simulink model "dvbs2hdlTransmitterCore"  (R2024b)
settings: Solver=FixedStepDiscrete  StartTime=0.0  StopTime=0  RelTol=1e-3
libraries: hdlsllib x105, simulink x41, dspsigops x7, commseqgen3 x5, whdlutilities x5, commhdlcrc x2, dsphdlfiltering2 x1, whdlmod x1
(part 3 of 5)

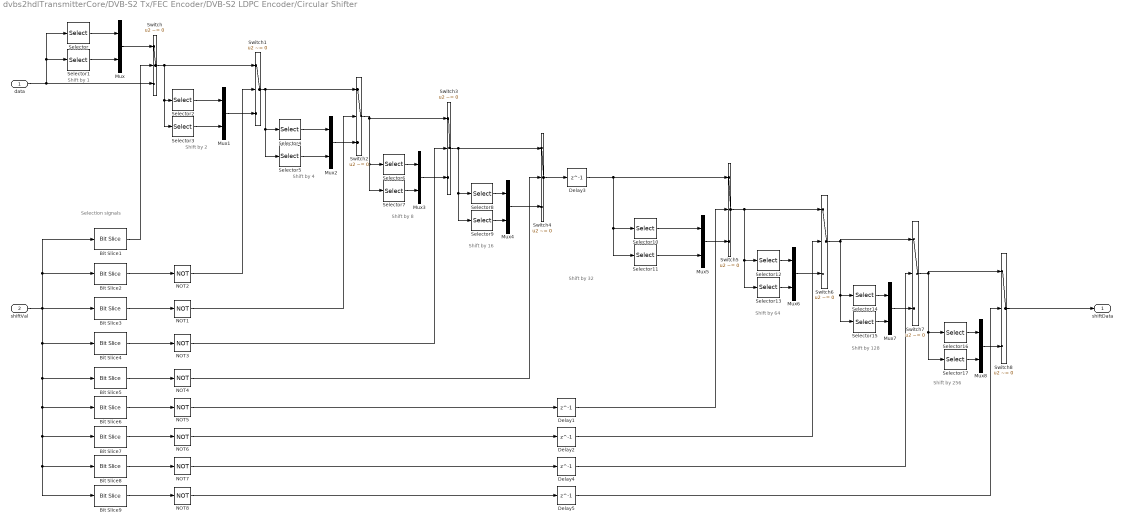
== system dvbs2hdlTransmitterCore/DVB-S2 Tx/FEC Encoder/DVB-S2 LDPC Encoder/Circular Shifter ==
  note: Shift by 256
  note: Shift by 128
  note: Shift by 64
  note: Shift by 32
  note: Shift by 16
  note: Shift by 8
  note: Shift by 4
  note: Shift by 2
  note: Shift by 1
  note: Selection signals
  data : Inport
  shiftVal : Inport  Port=2
  Bit Slice1 : hdlsllib/Logic and Bit Operations/Bit Slice  lidx=0  ridx=0
  Bit Slice2 : hdlsllib/Logic and Bit Operations/Bit Slice  lidx=1  ridx=1
  Bit Slice3 : hdlsllib/Logic and Bit Operations/Bit Slice  lidx=2  ridx=2
  Bit Slice4 : hdlsllib/Logic and Bit Operations/Bit Slice  lidx=3  ridx=3
  Bit Slice5 : hdlsllib/Logic and Bit Operations/Bit Slice  lidx=4  ridx=4
  Bit Slice6 : hdlsllib/Logic and Bit Operations/Bit Slice  lidx=5  ridx=5
  Bit Slice7 : hdlsllib/Logic and Bit Operations/Bit Slice  lidx=6  ridx=6
  Bit Slice8 : hdlsllib/Logic and Bit Operations/Bit Slice  lidx=7  ridx=7
  Bit Slice9 : hdlsllib/Logic and Bit Operations/Bit Slice  lidx=8  ridx=8
  Delay{1..5} (5 alike) : Delay  DelayLength=1
  Mux{,1..8} (9 alike) : Mux  Inputs=2
  NOT{1..8} (8 alike) : Logic  Operator=NOT  IconShape=distinctive  AllPortsSameDT=off  OutDataTypeStr=boolean
  Selector : Selector  InputPortWidth=360  IndexOptions=Index vector (dialog)  Indices=[2 : 360]  OutputSizes=1
  Selector1 : Selector  InputPortWidth=360  IndexOptions=Index vector (dialog)  Indices=[1]  OutputSizes=1
  Selector10 : Selector  InputPortWidth=360  IndexOptions=Index vector (dialog)  Indices=[33: 360]  OutputSizes=1
  Selector11 : Selector  InputPortWidth=360  IndexOptions=Index vector (dialog)  Indices=[1:32]  OutputSizes=1
  Selector12 : Selector  InputPortWidth=360  IndexOptions=Index vector (dialog)  Indices=[65: 360]  OutputSizes=1
  Selector13 : Selector  InputPortWidth=360  IndexOptions=Index vector (dialog)  Indices=[1:64]  OutputSizes=1
  Selector14 : Selector  InputPortWidth=360  IndexOptions=Index vector (dialog)  Indices=[129: 360]  OutputSizes=1
  Selector15 : Selector  InputPortWidth=360  IndexOptions=Index vector (dialog)  Indices=[1:128]  OutputSizes=1
  Selector16 : Selector  InputPortWidth=360  IndexOptions=Index vector (dialog)  Indices=[257: 360]  OutputSizes=1
  Selector17 : Selector  InputPortWidth=360  IndexOptions=Index vector (dialog)  Indices=[1:256]  OutputSizes=1
  Selector2 : Selector  InputPortWidth=360  IndexOptions=Index vector (dialog)  Indices=[3 : 360]  OutputSizes=1
  Selector3 : Selector  InputPortWidth=360  IndexOptions=Index vector (dialog)  Indices=[1:2]  OutputSizes=1
  Selector4 : Selector  InputPortWidth=360  IndexOptions=Index vector (dialog)  Indices=[5 : 360]  OutputSizes=1
  Selector5 : Selector  InputPortWidth=360  IndexOptions=Index vector (dialog)  Indices=[1:4]  OutputSizes=1
  Selector6 : Selector  InputPortWidth=360  IndexOptions=Index vector (dialog)  Indices=[9 : 360]  OutputSizes=1
  Selector7 : Selector  InputPortWidth=360  IndexOptions=Index vector (dialog)  Indices=[1:8]  OutputSizes=1
  Selector8 : Selector  InputPortWidth=360  IndexOptions=Index vector (dialog)  Indices=[17 : 360]  OutputSizes=1
  Selector9 : Selector  InputPortWidth=360  IndexOptions=Index vector (dialog)  Indices=[1:16]  OutputSizes=1
  Switch{,1..8} (9 alike) : Switch  Criteria=u2 ~= 0  InputSameDT=off
  shiftData : Outport
  wires:
  Delay5/1 -> Switch8/2
  Delay4/1 -> Switch7/2
  Delay2/1 -> Switch6/2
  Delay1/1 -> Switch5/2
  Delay3/1 -> Switch5/1, Selector10/1, Selector11/1
  NOT8/1 -> Delay5/1
  NOT7/1 -> Delay4/1
  NOT6/1 -> Delay2/1
  NOT5/1 -> Delay1/1
  Switch4/1 -> Delay3/1
  NOT4/1 -> Switch4/2
  NOT3/1 -> Switch3/2
  NOT1/1 -> Switch2/2
  NOT2/1 -> Switch1/2
  Bit Slice1/1 -> Switch/2
  Bit Slice9/1 -> NOT8/1
  Bit Slice8/1 -> NOT7/1
  Bit Slice7/1 -> NOT6/1
  Bit Slice6/1 -> NOT5/1
  Bit Slice5/1 -> NOT4/1
  Bit Slice4/1 -> NOT3/1
  Bit Slice3/1 -> NOT1/1
  Bit Slice2/1 -> NOT2/1
  Mux8/1 -> Switch8/3
  Switch7/1 -> Switch8/1, Selector17/1, Selector16/1
  Selector16/1 -> Mux8/1
  Selector17/1 -> Mux8/2
  Mux7/1 -> Switch7/3
  Selector15/1 -> Mux7/2
  Switch6/1 -> Switch7/1, Selector15/1, Selector14/1
  Selector14/1 -> Mux7/1
  Mux6/1 -> Switch6/3
  Switch5/1 -> Switch6/1, Selector13/1, Selector12/1
  Selector13/1 -> Mux6/2
  Selector12/1 -> Mux6/1
  Selector10/1 -> Mux5/1
  Mux5/1 -> Switch5/3
  Selector11/1 -> Mux5/2
  Mux4/1 -> Switch4/3
  Selector8/1 -> Mux4/1
  Switch3/1 -> Selector9/1, Selector8/1, Switch4/1
  Selector9/1 -> Mux4/2
  Mux3/1 -> Switch3/3
  Switch2/1 -> Switch3/1, Selector7/1, Selector6/1
  Selector7/1 -> Mux3/2
  Selector6/1 -> Mux3/1
  Switch1/1 -> Selector5/1, Selector4/1, Switch2/1
  Selector4/1 -> Mux2/1
  Mux2/1 -> Switch2/3
  Selector5/1 -> Mux2/2
  Mux1/1 -> Switch1/3
  Switch/1 -> Switch1/1, Selector2/1, Selector3/1
  Selector2/1 -> Mux1/1
  Selector3/1 -> Mux1/2
  Selector1/1 -> Mux/2
  Selector/1 -> Mux/1
  Mux/1 -> Switch/1
  data/1 -> Switch/3, Selector1/1, Selector/1
  shiftVal/1 -> Bit Slice9/1, Bit Slice8/1, Bit Slice7/1, Bit Slice6/1, Bit Slice5/1, Bit Slice4/1, Bit Slice3/1, Bit Slice2/1, Bit Slice1/1
  Switch8/1 -> shiftData/1

== system dvbs2hdlTransmitterCore/DVB-S2 Tx/FEC Encoder/DVB-S2 LDPC Encoder/Input RAM ==
  iwr_data : Inport  Partition=on  PartitionDimension=1  PartitionWidth=1  PartitionOffset=0
  iwr_addr : Inport  Port=2
  iwr_enb : Inport  Port=3  Partition=on  PartitionDimension=1  PartitionWidth=1  PartitionOffset=0
  ird_addr : Inport  Port=4
  For Each : ForEach  DisableCoverage=on
  Simple Dual Port RAM : hdlsllib/HDL RAMs/Simple Dual Port RAM  ram_size=8
  ird_data : Outport  ConcatenationDimension=1
  wires:
  Simple Dual Port RAM/1 -> ird_data/1
  iwr_data/1 -> Simple Dual Port RAM/1
  iwr_addr/1 -> Simple Dual Port RAM/2
  iwr_enb/1 -> Simple Dual Port RAM/3
  ird_addr/1 -> Simple Dual Port RAM/4

== system dvbs2hdlTransmitterCore/DVB-S2 Tx/FEC Encoder/DVB-S2 LDPC Encoder/Parity Address Generator ==
  note: shiftLUT = (parity length - (Parity bit address -
      | ramLUT))/qFactor)
  note: ramLUT = remainder (Parity bit address spcified
      | in standard, qFactor)
  note: columnLUT gives total number of columns
      | in each row of a parity bit addresses
  enb : Inport
  lutIdx : Inport  Port=2
  nRows : Inport  Port=3
  reset : Inport  Port=4
  AND : Logic  IconShape=distinctive  AllPortsSameDT=off  OutDataTypeStr=boolean
  AND1 : Logic  IconShape=distinctive  AllPortsSameDT=off  OutDataTypeStr=boolean
  AND2 : Logic  IconShape=distinctive  AllPortsSameDT=off  OutDataTypeStr=boolean
  Add : Sum  OutDataTypeStr=fixdt(0,11,0)
  Add1 : Sum  OutDataTypeStr=uint8
  Constant : Constant  OutDataTypeStr=uint8  SampleTime=-1
  Data Type Conversion : DataTypeConversion  OutDataTypeStr=fixdt(0,11,0)  SaturateOnIntegerOverflow=off  RndMeth=Floor
  Delay{1..8} (8 alike) : Delay  DelayLength=1
  Delay10 : Delay
  Delay9 : Delay
  OR : Logic  Operator=OR  IconShape=distinctive  AllPortsSameDT=off  OutDataTypeStr=boolean
  OR1 : Logic  Operator=OR  IconShape=distinctive  AllPortsSameDT=off  OutDataTypeStr=boolean
  Relational Operator : RelationalOperator  Operator===  OutDataTypeStr=boolean  RndMeth=Simplest  InputSameDT=off
  Relational Operator1 : RelationalOperator  Operator===  OutDataTypeStr=boolean  RndMeth=Simplest  InputSameDT=off
  columnCounter : hdlsllib/Sources/HDL Counter  CountType=Count limited  CountInit=1  CountStep=1  CountMax=31  CountFromType=Initial value  CountFrom=1  CountResetPort=on  CountLoadPort=off  CountEnbPort=on  CountDirPort=off  CountHitOutputPort=off  CountDataType=Unsigned  CountWordLen=5  CountFracLen=0  CountSampTime=1
  columnsLUT : Lookup_n-D  NumberOfTableDimensions=1  BreakpointsSpecification=Even spacing  BreakpointsForDimension1=[1:20]  BreakpointsForDimension1FirstPoint=0  Table=columnSum  InterpMethod=Flat  RemoveProtectionInput=on  InternalRulePriority=Speed  OutDataTypeStr=fixdt(0,5,0)  RndMeth=Simplest
  ramLUT : Lookup_n-D  BreakpointsSpecification=Even spacing  BreakpointsForDimension1=[1:20]  BreakpointsForDimension2=[1:8]  BreakpointsForDimension1FirstPoint=0  BreakpointsForDimension1DataTypeStr=fixdt(0,11,0)  BreakpointsForDimension2DataTypeStr=fixdt(0,8,0)  Table=uint8(ramLUT)  TableDataTypeStr=Inherit: Inherit from 'Table data'  InterpMethod=Flat  RemoveProtectionInput=on  InternalRulePriority=Speed  OutDataTypeStr=Inherit: Inherit from 'Table data'  RndMeth=Simplest
      settings: InputPortMap=u0,u1
  rowCounter : hdlsllib/Sources/HDL Counter  CountType=Count limited  CountInit=1  CountStep=1  CountMax=162  CountFromType=Initial value  CountFrom=1  CountResetPort=on  CountLoadPort=off  CountEnbPort=on  CountDirPort=off  CountHitOutputPort=off  CountDataType=Unsigned  CountWordLen=8  CountFracLen=0  CountSampTime=1
  shiftLUT : Lookup_n-D  BreakpointsSpecification=Even spacing  BreakpointsForDimension1=[1:20]  BreakpointsForDimension2=[1:8]  BreakpointsForDimension1FirstPoint=0  BreakpointsForDimension1DataTypeStr=fixdt(0,11,0)  BreakpointsForDimension2DataTypeStr=fixdt(0,8,0)  Table=fi(shiftLUT,0,9,0)  TableDataTypeStr=Inherit: Inherit from 'Table data'  InterpMethod=Flat  RemoveProtectionInput=on  InternalRulePriority=Speed  OutDataTypeStr=Inherit: Inherit from 'Table data'  RndMeth=Simplest
      settings: InputPortMap=u0,u1
  rdEnb : Outport
  shift : Outport  Port=2
  endEnc : Outport  Port=3
  parityAddr : Outport  Port=4
  wires:
  Data Type Conversion/1 -> Delay8/1
  Delay2/1 -> shiftLUT/1, ramLUT/1
  rowCounter/1 -> Add/2, Relational Operator1/1
  nRows/1 -> Relational Operator1/2
  [rstColCount] -> OR/1
  Delay3/1 -> [rstColCount]
  OR/1 -> columnCounter/1
  Delay4/1 -> [rstRowCount]
  OR1/1 -> rowCounter/1
  [rstRowCount] -> OR1/1
  reset/1 -> OR/2, OR1/2
  columnsLUT/1 -> Delay1/1
  Add/1 -> columnsLUT/1, Delay2/1
  shiftLUT/1 -> Delay5/1
  Delay5/1 -> shift/1
  lutIdx/1 -> Add/1
  Delay1/1 -> Relational Operator/2
  columnCounter/1 -> Relational Operator/1, Data Type Conversion/1
  AND/1 -> rowCounter/2
  [rstColCount] -> AND/2
  enb/1 -> Delay7/1, columnCounter/2, AND/1
  AND1/1 -> Delay10/1
  Relational Operator1/1 -> AND1/2
  ramLUT/1 -> Delay6/1
  Delay8/1 -> shiftLUT/2, ramLUT/2
  Relational Operator/1 -> AND2/1
  AND2/1 -> Delay9/1, AND1/1
  Delay7/1 -> AND2/2
  Delay9/1 -> Delay3/1, rdEnb/1
  Add1/1 -> parityAddr/1
  Delay6/1 -> Add1/2
  Constant/1 -> Add1/1
  Delay10/1 -> Delay4/1, endEnc/1

== system dvbs2hdlTransmitterCore/DVB-S2 Tx/FEC Encoder/DVB-S2 LDPC Encoder/Parity RAM ==
  pwr_data : Inport
  pwr_addr : Inport  Port=2
  pwr_enb : Inport  Port=3
  prd_addr : Inport  Port=4
  AND : Logic  IconShape=distinctive  AllPortsSameDT=off  OutDataTypeStr=boolean
  ConvertToMux : MATLAB Function  TreatAsAtomicUnit=on
  ConvertToWord : MATLAB Function  TreatAsAtomicUnit=on
  Data Type Conversion{,1..3} (4 alike) : DataTypeConversion  OutDataTypeStr=fixdt(0,1,0)  SaturateOnIntegerOverflow=off  RndMeth=Floor
  Delay : Delay  DelayLength=1
  Delay1 : Delay  DelayLength=1
  Dual Port RAM System{,1..3} (4 alike) : hdlsllib/HDL RAMs/Dual Port RAM System  RAMType=Simple dual port  AsyncRead=off  WriteOutputValue=New data  RAMInitialValue=0  allowBusInputs=off  WritesHaveOutput=on  NumReads=0  NumWrites=1  SimulateUsing=Code generation  ModelRAMDelay=on
  Mux : Mux
  Relational Operator : RelationalOperator  Operator===  OutDataTypeStr=boolean  RndMeth=Simplest  InputSameDT=off
  Selector : Selector  InputPortWidth=360  IndexOptions=Index vector (dialog)  Indices=[1:90]  OutputSizes=1
  Selector1 : Selector  InputPortWidth=360  IndexOptions=Index vector (dialog)  Indices=[91:180]  OutputSizes=1
  Selector2 : Selector  InputPortWidth=360  IndexOptions=Index vector (dialog)  Indices=[181:270]  OutputSizes=1
  Selector3 : Selector  InputPortWidth=360  IndexOptions=Index vector (dialog)  Indices=[271:360]  OutputSizes=1
  Switch : Switch  Criteria=u2 > Threshold  SaturateOnIntegerOverflow=off  InputSameDT=off
  prd_data : Outport
  wires:
  ConvertToMux/2(y2) -> Mux/2
  ConvertToMux/4(y4) -> Mux/4
  Dual Port RAM System2/1 -> ConvertToMux/4(u4)
  Dual Port RAM System/1 -> ConvertToMux/1(u1)
  Dual Port RAM System1/1 -> ConvertToMux/2(u2)
  ConvertToMux/1(y1) -> Mux/1
  ConvertToMux/3(y3) -> Mux/3
  Dual Port RAM System3/1 -> ConvertToMux/3(u3)
  Mux/1 -> Switch/3
  ConvertToWord/3(y3) -> Dual Port RAM System3/1
  Data Type Conversion2/1 -> ConvertToWord/3(u3)
  ConvertToWord/1(y1) -> Dual Port RAM System/1
  ConvertToWord/4(y4) -> Dual Port RAM System2/1
  Data Type Conversion3/1 -> ConvertToWord/4(u4)
  Selector3/1 -> Data Type Conversion3/1
  Selector1/1 -> Data Type Conversion1/1
  Data Type Conversion/1 -> ConvertToWord/1(u1)
  ConvertToWord/2(y2) -> Dual Port RAM System1/1
  pwr_data/1 -> Selector/1, Selector1/1, Selector2/1, Selector3/1, Delay/1
  Selector2/1 -> Data Type Conversion2/1
  Selector/1 -> Data Type Conversion/1
  Data Type Conversion1/1 -> ConvertToWord/2(u2)
  Switch/1 -> prd_data/1
  pwr_addr/1 -> Dual Port RAM System/2, Dual Port RAM System1/2, Dual Port RAM System2/2, Dual Port RAM System3/2, Relational Operator/1
  pwr_enb/1 -> Dual Port RAM System/3, Dual Port RAM System1/3, Dual Port RAM System3/3, Dual Port RAM System2/3, Delay1/1
  prd_addr/1 -> Dual Port RAM System/4, Relational Operator/2, Dual Port RAM System1/4, Dual Port RAM System3/4, Dual Port RAM System2/4
  Delay/1 -> Switch/1
  AND/1 -> Switch/2
  Relational Operator/1 -> AND/1
  Delay1/1 -> AND/2

== system dvbs2hdlTransmitterCore/DVB-S2 Tx/Interleaver/DVB-S2 HDL Interleaver/RAM ==
  wr_din : Inport
  wr_addr : Inport  Port=2
  wr_en : Inport  Port=3
  rd_addr : Inport  Port=4
  rd_valid : Inport  Port=5
  rd_end : Inport  Port=6
  rd_start : Inport  Port=7
  Delay : Delay  DelayLength=1
  Delay1 : Delay  DelayLength=1
  Delay{3..13} (11 alike) : Delay
  Delay2 : Delay  DelayLength=1
  Single RAM Using Two RAMs : Subsystem
  Wrap Address : Subsystem
  rd_dout : Outport
  rd_startOut : Outport  Port=2
  rd_endOut : Outport  Port=3
  rd_validOut : Outport  Port=4
  wires:
  Single RAM Using Two RAMs/1(rd_dout) -> Delay9/1
  Delay8/1 -> Single RAM Using Two RAMs/4(rd_addr)
  Delay7/1 -> Single RAM Using Two RAMs/3(wr_en)
  Delay6/1 -> Single RAM Using Two RAMs/2(wr_addr)
  Delay12/1 -> Single RAM Using Two RAMs/1(wr_din)
  wr_en/1 -> Delay7/1
  wr_din/1 -> Delay12/1
  wr_addr/1 -> Delay6/1
  rd_valid/1 -> Delay3/1
  Delay/1 -> Delay10/1
  rd_start/1 -> Delay4/1
  rd_end/1 -> Delay5/1
  Delay1/1 -> Delay11/1
  Delay2/1 -> Delay13/1
  rd_addr/1 -> Wrap Address/1(u)
  Wrap Address/1(y) -> Delay8/1
  Delay3/1 -> Delay/1
  Delay4/1 -> Delay1/1
  Delay5/1 -> Delay2/1
  Delay9/1 -> rd_dout/1
  Delay10/1 -> rd_validOut/1
  Delay11/1 -> rd_startOut/1
  Delay13/1 -> rd_endOut/1

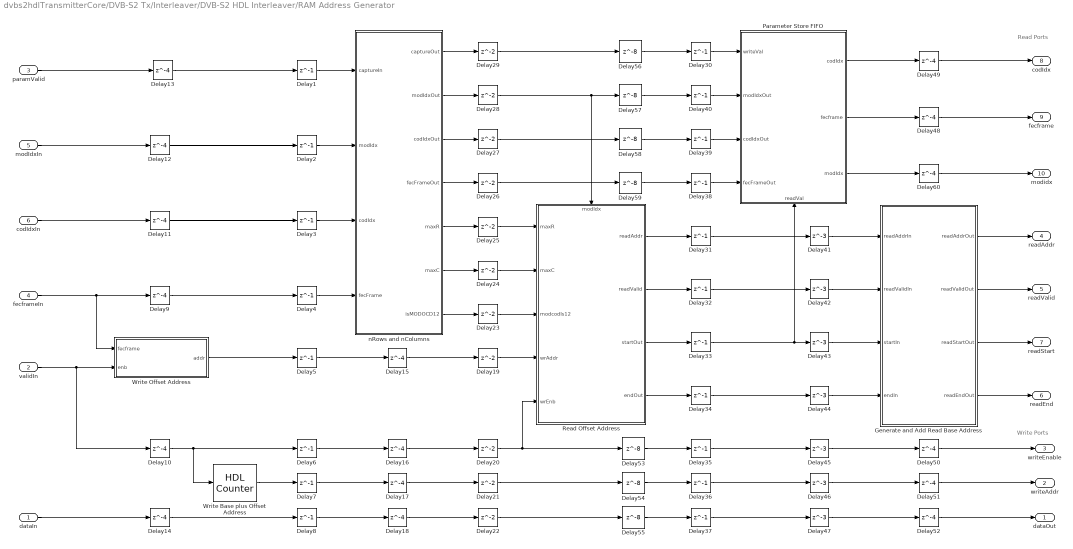
== system dvbs2hdlTransmitterCore/DVB-S2 Tx/Interleaver/DVB-S2 HDL Interleaver/RAM Address Generator ==
  note: Read Ports
  note: Write Ports
  dataIn : Inport
  validIn : Inport  Port=2
  paramValid : Inport  Port=3
  fecframeIn : Inport  Port=4
  modIdxIn : Inport  Port=5
  codIdxIn : Inport  Port=6
  Delay{1..8,30..40} (19 alike) : Delay  DelayLength=1
  Delay{9..18,48..52,60} (16 alike) : Delay  DelayLength=4
  Delay{19..29} (11 alike) : Delay
  Delay{41..47} (7 alike) : Delay  DelayLength=3
  Delay{53..59} (7 alike) : Delay  DelayLength=8
  Generate and Add Read Base Address : Subsystem
  Parameter Store FIFO : Subsystem
      settings: PortSchema="{\"entries\":[{\"content\":{\"sides\":[{\"content\":{\"connectorIds\":[\"In1\",\"In2\",\"In3\",\"In4\"]},\"type\":\"ConnectorPlacement.EquallySpacedRectSide\",\"uuid\":\"6d8768ca-7228-4729-bdbf-9ebbcab1a5aa\"},{\"content\":{\"connectorIds\":[\"Out1\",\"Out2\",\"Out3\"],\"side\":\"RIGHT\"},\"type\":\"ConnectorPlacement.EquallySpacedRectSide\",\"uuid\":\"b8ba0d5a-2b82-4d8d-a9c2-2d3fcacc6c9a\"},{\"content\":{\"connectorIds\":[],\"side\":\"TOP\"},\"type\":\"ConnectorPlacement.EquallySpacedRectSide\",\"uuid\":\"1722486f-4cf2-41b6-8f78-86c27924cee8\"},{\"content\":{\"connectorIds\":[\"In5\"],\"side\":\"BOTTOM\"},\"type\":\"ConnectorPlacement.EquallySpacedRectSide\",\"uuid\":\"409cf5cf-743f-45fc-b63a-6af4afdbc038\"}]},\"type\":\"ConnectorPlacement.EquallySpacedConnector\",\"uuid\":\"90aa5513-49d5-48a8-89f8-bb5993d63f9c\"}],\"packageUris\":[\"http://schema.mathworks.com/mf0/Connector/R2020b\"],\"version\":\"1.0\"}"
  Read Offset Address : Subsystem
      settings: PortSchema="{\"entries\":[{\"content\":{\"sides\":[{\"content\":{\"connectorIds\":[\"In1\",\"In2\",\"In3\",\"In4\",\"In5\"]},\"type\":\"ConnectorPlacement.EquallySpacedRectSide\",\"uuid\":\"5402c4dc-a10b-48e3-8f95-7f847805ec5d\"},{\"content\":{\"connectorIds\":[\"Out1\",\"Out2\",\"Out3\",\"Out4\"],\"side\":\"RIGHT\"},\"type\":\"ConnectorPlacement.EquallySpacedRectSide\",\"uuid\":\"8a6cd6fa-14b0-4c5b-9941-8705d53d88ec\"},{\"content\":{\"connectorIds\":[\"In6\"],\"side\":\"TOP\"},\"type\":\"ConnectorPlacement.EquallySpacedRectSide\",\"uuid\":\"b3c4ffa4-8fdb-4990-82df-071a871880c5\"}]},\"type\":\"ConnectorPlacement.EquallySpacedConnector\",\"uuid\":\"ded72292-2df4-4b7d-a4b9-106fb997de76\"}],\"packageUris\":[\"http://schema.mathworks.com/mf0/Connector/R2020b\"],\"version\":\"1.0\"}"
  Write Base plus Offset Address : hdlsllib/Sources/HDL Counter  CountType=Count limited  CountInit=0  CountStep=1  CountMax=ConfigRx.RAMCapacity - 1  CountFromType=Initial value  CountFrom=0  CountResetPort=off  CountLoadPort=off  CountEnbPort=on  CountDirPort=off  CountHitOutputPort=off  CountDataType=Unsigned  CountWordLen=nextpow2(ConfigRx.RAMCapacity - 1)  CountFracLen=0  CountSampTime=1
  Write Offset Address : Subsystem
  nRows and nColumns : Subsystem
  dataOut : Outport
  writeAddr : Outport  Port=2
  writeEnable : Outport  Port=3
  readAddr : Outport  Port=4
  readValid : Outport  Port=5
  readEnd : Outport  Port=6
  readStart : Outport  Port=7
  codIdx : Outport  Port=8
  fecframe : Outport  Port=9
  modidx : Outport  Port=10
  wires:
  paramValid/1 -> Delay13/1
  Delay60/1 -> modidx/1
  Parameter Store FIFO/3(modIdx) -> Delay60/1
  nRows and nColumns/5(maxR) -> Delay25/1
  validIn/1 -> Write Offset Address/2(enb), Delay10/1
  nRows and nColumns/6(maxC) -> Delay24/1
  Write Base plus Offset Address/1 -> Delay7/1
  modIdxIn/1 -> Delay12/1
  fecframeIn/1 -> Delay9/1, Write Offset Address/1(fecframe)
  nRows and nColumns/7(isMODOCD12) -> Delay23/1
  codIdxIn/1 -> Delay11/1
  dataIn/1 -> Delay14/1
  Generate and Add Read Base Address/1(readAddrOut) -> readAddr/1
  Generate and Add Read Base Address/2(readValidOut) -> readValid/1
  Generate and Add Read Base Address/3(readStartOut) -> readStart/1
  Generate and Add Read Base Address/4(readEndOut) -> readEnd/1
  Write Offset Address/1(addr) -> Delay5/1
  nRows and nColumns/3(codIdxOut) -> Delay27/1
  nRows and nColumns/4(fecFrameOut) -> Delay26/1
  nRows and nColumns/1(captureOut) -> Delay29/1
  Parameter Store FIFO/1(codIdx) -> Delay49/1
  Parameter Store FIFO/2(fecframe) -> Delay48/1
  nRows and nColumns/2(modIdxOut) -> Delay28/1
  Delay2/1 -> nRows and nColumns/2(modIdx)
  Delay3/1 -> nRows and nColumns/3(codIdx)
  Delay4/1 -> nRows and nColumns/4(fecFrame)
  Delay5/1 -> Delay15/1
  Delay6/1 -> Delay16/1
  Delay7/1 -> Delay17/1
  Delay9/1 -> Delay4/1
  Delay10/1 -> Write Base plus Offset Address/1, Delay6/1
  Delay11/1 -> Delay3/1
  Delay12/1 -> Delay2/1
  Delay8/1 -> Delay18/1
  Delay14/1 -> Delay8/1
  Delay13/1 -> Delay1/1
  Delay1/1 -> nRows and nColumns/1(captureIn)
  Delay15/1 -> Delay19/1
  Delay16/1 -> Delay20/1
  Delay17/1 -> Delay21/1
  Delay18/1 -> Delay22/1
  Delay20/1 -> Read Offset Address/5(wrEnb), Delay53/1
  Delay21/1 -> Delay54/1
  Delay22/1 -> Delay55/1
  Delay26/1 -> Delay59/1
  Delay27/1 -> Delay58/1
  Delay28/1 -> Read Offset Address/6(modIdx), Delay57/1
  Delay29/1 -> Delay56/1
  Delay30/1 -> Parameter Store FIFO/1(writeVal)
  Delay31/1 -> Delay41/1
  Delay32/1 -> Delay42/1
  Delay33/1 -> Delay43/1, Parameter Store FIFO/5(readVal)
  Delay34/1 -> Delay44/1
  Delay35/1 -> Delay45/1
  Delay36/1 -> Delay46/1
  Delay37/1 -> Delay47/1
  Delay38/1 -> Parameter Store FIFO/4(fecFrameOut)
  Delay39/1 -> Parameter Store FIFO/3(codIdxOut)
  Delay40/1 -> Parameter Store FIFO/2(modIdxOut)
  Delay41/1 -> Generate and Add Read Base Address/1(readAddrIn)
  Delay42/1 -> Generate and Add Read Base Address/2(readValidIn)
  Delay43/1 -> Generate and Add Read Base Address/3(startIn)
  Delay44/1 -> Generate and Add Read Base Address/4(endIn)
  Delay45/1 -> Delay50/1
  Delay46/1 -> Delay51/1
  Delay47/1 -> Delay52/1
  Delay48/1 -> fecframe/1
  Delay49/1 -> codIdx/1
  Delay50/1 -> writeEnable/1
  Delay51/1 -> writeAddr/1
  Delay52/1 -> dataOut/1
  Delay53/1 -> Delay35/1
  Delay54/1 -> Delay36/1
  Delay55/1 -> Delay37/1
  Delay59/1 -> Delay38/1
  Delay58/1 -> Delay39/1
  Delay57/1 -> Delay40/1
  Delay56/1 -> Delay30/1
  Delay25/1 -> Read Offset Address/1(maxR)
  Delay24/1 -> Read Offset Address/2(maxC)
  Delay23/1 -> Read Offset Address/3(modcodIs12)
  Delay19/1 -> Read Offset Address/4(wrAddr)
  Read Offset Address/1(readAddr) -> Delay31/1
  Read Offset Address/2(readValid) -> Delay32/1
  Read Offset Address/3(startOut) -> Delay33/1
  Read Offset Address/4(endOut) -> Delay34/1

== system dvbs2hdlTransmitterCore/DVB-S2 Tx/PL Frame Generator/Multiplexer/No HDL ==
  In1 : Inport
  In2 : Inport  Port=2
  In5 : Inport  Port=3
  dummyValid : Inport  Port=4
  Assertion : Assertion
  Assertion1 : Assertion
  Delay : Delay  DelayLength=5  InitialCondition=1
  Delay1 : Delay  DelayLength=5  InitialCondition=1
  Logical Operator{,1,3,5} (4 alike) : Logic  AllPortsSameDT=off  OutDataTypeStr=boolean
  Logical Operator2 : Logic  Operator=NOT  Inputs=3  AllPortsSameDT=off  OutDataTypeStr=boolean
  Logical Operator4 : Logic  Operator=OR  Inputs=3  AllPortsSameDT=off  OutDataTypeStr=boolean
  Logical Operator6 : Logic  Operator=NOT  AllPortsSameDT=off  OutDataTypeStr=boolean
  wires:
  Delay1/1 -> Assertion1/1
  Delay/1 -> Assertion/1
  Logical Operator6/1 -> Delay1/1
  Logical Operator5/1 -> Logical Operator6/1
  dummyValid/1 -> Logical Operator5/2
  Logical Operator2/1 -> Delay/1
  In2/1 -> Logical Operator3/1, Logical Operator/2
  Logical Operator4/1 -> Logical Operator2/1, Logical Operator5/1
  Logical Operator3/1 -> Logical Operator4/3
  Logical Operator1/1 -> Logical Operator4/2
  Logical Operator/1 -> Logical Operator4/1
  In5/1 -> Logical Operator3/2, Logical Operator1/2
  In1/1 -> Logical Operator1/1, Logical Operator/1

== system dvbs2hdlTransmitterCore/DVB-S2 Tx/PL Frame Generator/PL Data Scrambler/PL Scrambler Gold Sequence Generator ==
  reset : Inport
  validIn : Inport  Port=2
  Bit Concat : hdlsllib/Logic and Bit Operations/Bit Concat  numInputs=2
  Delay{,3..4,10,12..15} (8 alike) : Delay  DelayLength=1
  Delay{1..2,5..9,11} (8 alike) : Delay
  Logical Operator : Logic  Operator=XOR  AllPortsSameDT=off  OutDataTypeStr=boolean
  Logical Operator1 : Logic  Operator=XOR  AllPortsSameDT=off  OutDataTypeStr=boolean
  Logical Operator2 : Logic  Operator=OR  AllPortsSameDT=off  OutDataTypeStr=boolean
  Subsystem : Subsystem
  dataOut : Outport
  validOut : Outport  Port=2
  wires:
  Logical Operator2/1 -> Delay1/1
  Subsystem/4(yM0) -> Delay9/1
  Subsystem/3(xMn) -> Delay8/1
  Subsystem/2(yM131072) -> Delay7/1
  Subsystem/1(xMnp131072) -> Delay6/1
  reset/1 -> Delay3/1
  Bit Concat/1 -> Delay14/1
  Logical Operator/1 -> Delay12/1
  Logical Operator1/1 -> Delay10/1
  validIn/1 -> Delay4/1
  Delay/1 -> Delay11/1, Logical Operator2/2
  Delay11/1 -> Subsystem/1(reset)
  Delay1/1 -> Subsystem/Enable
  Delay2/1 -> Delay5/1
  Delay3/1 -> Delay/1
  Delay4/1 -> Logical Operator2/1, Delay2/1
  Delay5/1 -> Delay13/1
  Delay6/1 -> Logical Operator1/1
  Delay7/1 -> Logical Operator1/2
  Delay8/1 -> Logical Operator/1
  Delay9/1 -> Logical Operator/2
  Delay10/1 -> Bit Concat/1
  Delay12/1 -> Bit Concat/2
  Delay13/1 -> Delay15/1
  Delay14/1 -> dataOut/1
  Delay15/1 -> validOut/1

== system dvbs2hdlTransmitterCore/DVB-S2 Tx/PL Frame Generator/PL Header Generator/PL Header Bits Generator ==
  trigger : Inport
  pilotActive : Inport  Port=2
  modcod : Inport  Port=3
  fecframe : Inport  Port=4
  Data Type Conversion : DataTypeConversion  OutDataTypeStr=fixdt(0,1,0)  SaturateOnIntegerOverflow=off  RndMeth=Floor
  Data Type Conversion2 : DataTypeConversion  OutDataTypeStr=boolean  SaturateOnIntegerOverflow=off  RndMeth=Floor
  Header Bits Packer : MATLAB Function  TreatAsAtomicUnit=on
  Multiport Switch : MultiPortSwitch  DataPortOrder=Zero-based contiguous  Inputs=2  zeroidx=on  SaturateOnIntegerOverflow=off  InputSameDT=off
  Multiport Switch1 : MultiPortSwitch  DataPortOrder=Zero-based contiguous  Inputs=2  zeroidx=on  SaturateOnIntegerOverflow=off  InputSameDT=off
  PLSC Generator : Subsystem
  SOF Generator : Subsystem
      settings: PortSchema="{\"entries\":[{\"content\":{\"sides\":[{\"content\":{\"connectorIds\":[\"In1\"]},\"type\":\"ConnectorPlacement.EquallySpacedRectSide\",\"uuid\":\"a29cb59e-7642-4586-acf2-97c3dde01fe7\"},{\"content\":{\"connectorIds\":[\"Out1\",\"Out2\"],\"side\":\"RIGHT\"},\"type\":\"ConnectorPlacement.EquallySpacedRectSide\",\"uuid\":\"b2f13b17-be8b-4be3-ae05-864d033eb7d5\"},{\"content\":{\"connectorIds\":[\"Out3\"],\"side\":\"TOP\"},\"type\":\"ConnectorPlacement.EquallySpacedRectSide\",\"uuid\":\"d91dbfe1-ee73-468c-8f85-3881ff3ec8ca\"}]},\"type\":\"ConnectorPlacement.EquallySpacedConnector\",\"uuid\":\"e82ac009-3a14-4756-89bb-1c258ae23586\"}],\"packageUris\":[\"http://schema.mathworks.com/mf0/Connector/R2020b\"],\"version\":\"1.0\"}"
  bitsOut : Outport
  bitsStart : Outport  Port=2
  bitsEnd : Outport  Port=3
  bitsValid : Outport  Port=4
  wires:
  PLSC Generator/3(endOfPLSC) -> bitsEnd/1
  SOF Generator/3(startOfSOF) -> bitsStart/1
  SOF Generator/2(validOut) -> Multiport Switch1/2
  Multiport Switch1/1 -> bitsValid/1
  Multiport Switch/1 -> bitsOut/1
  pilotActive/1 -> Header Bits Packer/2(pilotActive)
  SOF Generator/1(dataOut) -> Multiport Switch/2
  fecframe/1 -> Data Type Conversion/1
  Header Bits Packer/3(start) -> PLSC Generator/3(bitsStart)
  Data Type Conversion2/1 -> PLSC Generator/2(bits1to6)
  modcod/1 -> Header Bits Packer/3(modcod)
  PLSC Generator/1(bitsOut) -> Multiport Switch/3
  Data Type Conversion/1 -> Header Bits Packer/4(fecframe)
  Header Bits Packer/2(bits1to6) -> Data Type Conversion2/1
  Header Bits Packer/4(valid) -> PLSC Generator/4(bitsValidIn)
  PLSC Generator/2(bitsValid) -> Multiport Switch/1, Multiport Switch1/3, Multiport Switch1/1
  trigger/1 -> SOF Generator/1(trigger), Header Bits Packer/1(trigger)
  Header Bits Packer/1(bit7) -> PLSC Generator/1(bit7)

== system dvbs2hdlTransmitterCore/DVB-S2 Tx/PL Frame Generator/PL Header Generator/piby2 BPSK Modulator ==
  bitsIn : Inport
  startIn : Inport  Port=2
  endIn : Inport  Port=3
  validIn : Inport  Port=4
  Constant1 : Constant  Value=exp(-1i*3*pi/4)  OutDataTypeStr=fixdt(1,18,16)  SampleTime=1/(Rsym)
      mask init:
      | Simulink.suppressDiagnostic(gcb, 'SimulinkFixedPoint:util:fxpParameterPrecisionLoss');
  Constant2 : Constant  Value=exp(1i*pi/4)  OutDataTypeStr=fixdt(1,18,16)  SampleTime=1/(Rsym)
      mask init:
      | Simulink.suppressDiagnostic(gcb, 'SimulinkFixedPoint:util:fxpParameterPrecisionLoss');
  Data Type Conversion : DataTypeConversion  OutDataTypeStr=boolean  SaturateOnIntegerOverflow=off  RndMeth=Floor
  Delay{1..2,4..5} (4 alike) : Delay  DelayLength=1
  Extract Bits : simulink/Logic and Bit Operations/Extract Bits  bitsToExtract=Range of bits  numBits=8  bitIdxRange=0  outScalingMode=Treat bit field as an integer
  Gain : Gain  Gain=exp(1i*pi/2)  ParamDataTypeStr=fixdt(1,16,14)  OutDataTypeStr=Inherit: Same as input
      mask init:
      | Simulink.suppressDiagnostic(gcb, 'SimulinkFixedPoint:util:fxpParameterPrecisionLoss');
  HDL Counter : hdlsllib/Sources/HDL Counter  CountType=Count limited  CountInit=0  CountStep=1  CountMax=90 - 1  CountFromType=Initial value  CountFrom=0  CountResetPort=on  CountLoadPort=off  CountEnbPort=on  CountDirPort=off  CountHitOutputPort=off  CountDataType=Unsigned  CountWordLen=nextpow2(90 - 1)  CountFracLen=0  CountSampTime=1
  Switch : Switch  Criteria=u2 ~= 0  SaturateOnIntegerOverflow=off  InputSameDT=off
  Switch1 : Switch  Criteria=u2 ~= 0  SaturateOnIntegerOverflow=off  InputSameDT=off
  dataOut : Outport
  startOut : Outport  Port=2
  endOut : Outport  Port=3
  validOut : Outport  Port=4
  wires:
  Delay2/1 -> startOut/1
  Delay4/1 -> validOut/1, HDL Counter/2
  Delay1/1 -> endOut/1
  endIn/1 -> Delay1/1
  Gain/1 -> Switch1/1
  Switch/1 -> Gain/1, Switch1/3
  Switch1/1 -> dataOut/1
  Data Type Conversion/1 -> Switch1/2
  HDL Counter/1 -> Extract Bits/1
  Extract Bits/1 -> Data Type Conversion/1
  Constant2/1 -> Switch/3
  Constant1/1 -> Switch/1
  startIn/1 -> HDL Counter/1, Delay2/1
  validIn/1 -> Delay4/1
  Delay5/1 -> Switch/2
  bitsIn/1 -> Delay5/1

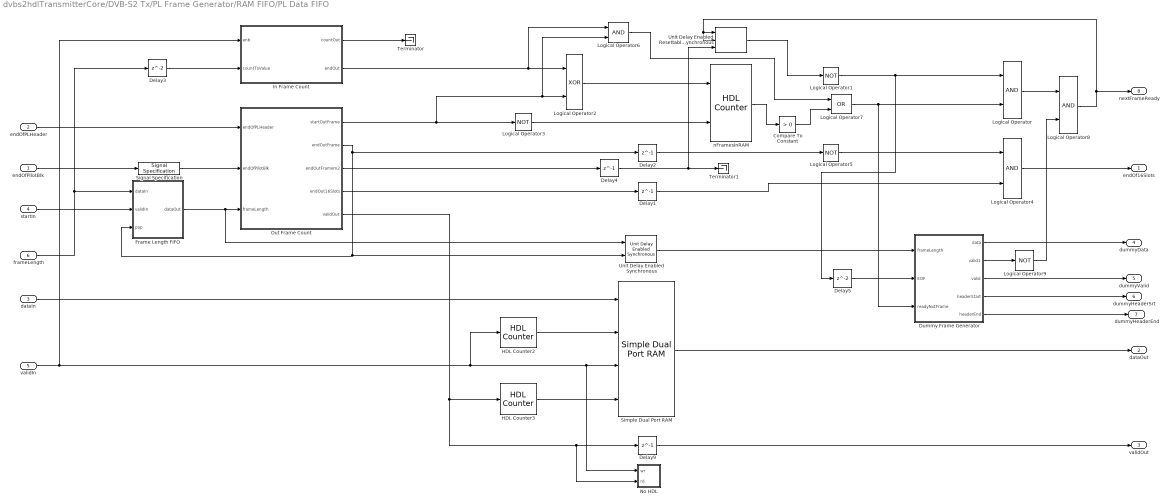
== system dvbs2hdlTransmitterCore/DVB-S2 Tx/PL Frame Generator/RAM FIFO/PL Data FIFO ==
  endOfPilotBlk : Inport
  endOfPLHeader : Inport  Port=2
  dataIn : Inport  Port=3
  startIn : Inport  Port=4
  validIn : Inport  Port=5
  frameLength : Inport  Port=6
  Compare To Constant : simulink/Logic and Bit Operations/Compare To Constant  relop=>  const=0  OutDataTypeStr=boolean
  Delay{1..2,4,9} (4 alike) : Delay  DelayLength=1
  Delay3 : Delay
  Delay5 : Delay
  Dummy Frame Generator : Subsystem
  Frame Length FIFO : Subsystem
  HDL Counter2 : hdlsllib/Sources/HDL Counter  CountType=Count limited  CountInit=0  CountStep=1  CountMax=2^16-1  CountFromType=Initial value  CountFrom=0  CountResetPort=off  CountLoadPort=off  CountEnbPort=on  CountDirPort=off  CountHitOutputPort=off  CountDataType=Unsigned  CountWordLen=16  CountFracLen=0  CountSampTime=1
  HDL Counter3 : hdlsllib/Sources/HDL Counter  CountType=Count limited  CountInit=0  CountStep=1  CountMax=2^16-1  CountFromType=Initial value  CountFrom=0  CountResetPort=off  CountLoadPort=off  CountEnbPort=on  CountDirPort=off  CountHitOutputPort=off  CountDataType=Unsigned  CountWordLen=16  CountFracLen=0  CountSampTime=1
  In Frame Count : MATLAB Function  TreatAsAtomicUnit=on
  Logical Operator{,4,6,8} (4 alike) : Logic  AllPortsSameDT=off  OutDataTypeStr=boolean
  Logical Operator{1,3,5,9} (4 alike) : Logic  Operator=NOT  AllPortsSameDT=off  OutDataTypeStr=boolean
  Logical Operator2 : Logic  Operator=XOR  AllPortsSameDT=off  OutDataTypeStr=boolean
  Logical Operator7 : Logic  Operator=OR  AllPortsSameDT=off  OutDataTypeStr=boolean
  No HDL : Subsystem
  Out Frame Count : MATLAB Function  TreatAsAtomicUnit=on
  Signal Specification : SignalSpecification  OutDataTypeStr=boolean
  Simple Dual Port RAM : hdlsllib/HDL RAMs/Simple Dual Port RAM  ram_size=16
  Terminator : Terminator
  Terminator1 : Terminator
  Unit Delay Enabled Synchronous : hdlsllib/Discrete/Unit Delay Enabled Synchronous  InitialCondition=0.0  SampleTime=-1
  Unit Delay Enabled Resettable Synchronous : hdlsllib/Discrete/Unit Delay Enabled Resettable Synchronous  InitialCondition=0.0  SampleTime=-1
  nFramesInRAM : hdlsllib/Sources/HDL Counter  CountType=Free running  CountInit=0  CountStep=1  CountMax=25  CountFromType=Initial value  CountFrom=0  CountResetPort=off  CountLoadPort=off  CountEnbPort=on  CountDirPort=on  CountHitOutputPort=off  CountDataType=Unsigned  CountWordLen=8  CountFracLen=0  CountSampTime=1
  endOf16Slots : Outport
  dataOut : Outport  Port=2
  validOut : Outport  Port=3
  dummyData : Outport  Port=4
  dummyValid : Outport  Port=5
  dummyHeaderSrt : Outport  Port=6
  dummyHeaderEnd : Outport  Port=7
  nextFrameReady : Outport  Port=8
  wires:
  Delay5/1 -> Dummy Frame Generator/2(EOF)
  Delay4/1 -> Terminator1/1, Unit Delay Enabled Resettable Synchronous/3
  Out Frame Count/3(endOutFramem2) -> Delay4/1
  Dummy Frame Generator/5(headerEnd) -> dummyHeaderEnd/1
  Dummy Frame Generator/4(headerStart) -> dummyHeaderSrt/1
  Dummy Frame Generator/2(valid1) -> Logical Operator9/1
  Logical Operator9/1 -> Logical Operator8/2
  Logical Operator/1 -> Logical Operator8/1
  Logical Operator7/1 -> Dummy Frame Generator/3(readyNxtFrame), Logical Operator/2
  Dummy Frame Generator/3(valid) -> dummyValid/1
  Dummy Frame Generator/1(data) -> dummyData/1
  Unit Delay Enabled Synchronous/1 -> Dummy Frame Generator/1(frameLength)
  Out Frame Count/2(endOutFrame) -> Delay2/1, Unit Delay Enabled Synchronous/2, Frame Length FIFO/3(pop)
  Delay3/1 -> In Frame Count/2(countToValue)
  Logical Operator6/1 -> Logical Operator7/1
  Logical Operator5/1 -> Logical Operator4/1
  Logical Operator4/1 -> endOf16Slots/1
  Delay1/1 -> Logical Operator4/2
  Signal Specification/1 -> Out Frame Count/2(endOfPilotBlk)
  endOfPilotBlk/1 -> Signal Specification/1
  Frame Length FIFO/1(dataOut) -> Out Frame Count/3(frameLength), Unit Delay Enabled Synchronous/1
  startIn/1 -> Frame Length FIFO/2(validIn)
  Logical Operator8/1 -> nextFrameReady/1, Unit Delay Enabled Resettable Synchronous/1, Unit Delay Enabled Resettable Synchronous/2
  Delay9/1 -> validOut/1
  Simple Dual Port RAM/1 -> dataOut/1
  Logical Operator1/1 -> Logical Operator/1, Delay5/1
  Unit Delay Enabled Resettable Synchronous/1 -> Logical Operator1/1
  Delay2/1 -> Logical Operator5/1
  Compare To Constant/1 -> Logical Operator7/2
  Logical Operator3/1 -> nFramesInRAM/2
  nFramesInRAM/1 -> Compare To Constant/1
  Logical Operator2/1 -> nFramesInRAM/1
  In Frame Count/1(countOut) -> Terminator/1
  In Frame Count/2(endOut) -> Logical Operator2/1, Logical Operator6/1
  Out Frame Count/1(startOutFrame) -> Logical Operator2/2, Logical Operator6/2, Logical Operator3/1
  endOfPLHeader/1 -> Out Frame Count/1(endOfPLHeader)
  frameLength/1 -> Frame Length FIFO/1(dataIn), Delay3/1
  Out Frame Count/4(endOut16Slots) -> Delay1/1
  dataIn/1 -> Simple Dual Port RAM/1
  HDL Counter3/1 -> Simple Dual Port RAM/4
  validIn/1 -> In Frame Count/1(enb), HDL Counter2/1, No HDL/1(wr), Simple Dual Port RAM/3
  Out Frame Count/5(validOut) -> HDL Counter3/1, No HDL/2(rd), Delay9/1
  HDL Counter2/1 -> Simple Dual Port RAM/2

== system dvbs2hdlTransmitterCore/DVB-S2 Tx/PL Frame Generator/RAM FIFO/PL Header FIFO ==
  dataIn : Inport
  validIn : Inport  Port=2
  nextFrameReady : Inport  Port=3
  90x : MATLAB Function  TreatAsAtomicUnit=on
  Delay{1..3,9} (4 alike) : Delay  DelayLength=1
  HDL Counter2 : hdlsllib/Sources/HDL Counter  CountType=Count limited  CountInit=0  CountStep=1  CountMax=2^9 - 1  CountFromType=Initial value  CountFrom=0  CountResetPort=off  CountLoadPort=off  CountEnbPort=on  CountDirPort=off  CountHitOutputPort=off  CountDataType=Unsigned  CountWordLen=nextpow2(450)  CountFracLen=0  CountSampTime=1
  HDL Counter3 : hdlsllib/Sources/HDL Counter  CountType=Count limited  CountInit=0  CountStep=1  CountMax=2^9 - 1  CountFromType=Initial value  CountFrom=0  CountResetPort=off  CountLoadPort=off  CountEnbPort=on  CountDirPort=off  CountHitOutputPort=off  CountDataType=Unsigned  CountWordLen=nextpow2(450)  CountFracLen=0  CountSampTime=1
  No HDL : Subsystem
  Simple Dual Port RAM : hdlsllib/HDL RAMs/Simple Dual Port RAM  ram_size=nextpow2(450)
  dataOut : Outport
  startOut : Outport  Port=2
  endOut : Outport  Port=3
  validOut : Outport  Port=4
  endOut1 : Outport  Port=5
  wires:
  90x/4(endOutm1) -> Delay3/1
  Delay3/1 -> endOut1/1
  Delay2/1 -> endOut/1
  Delay1/1 -> startOut/1
  Delay9/1 -> validOut/1
  Simple Dual Port RAM/1 -> dataOut/1
  nextFrameReady/1 -> 90x/1(trigger)
  90x/3(endOut) -> Delay2/1
  90x/2(startOut) -> Delay1/1
  90x/1(validOut) -> Delay9/1, No HDL/2(rd), HDL Counter3/1
  HDL Counter2/1 -> Simple Dual Port RAM/2
  dataIn/1 -> Simple Dual Port RAM/1
  HDL Counter3/1 -> Simple Dual Port RAM/4
  validIn/1 -> No HDL/1(wr), HDL Counter2/1, Simple Dual Port RAM/3

== system dvbs2hdlTransmitterCore/DVB-S2 Tx/PL Frame Generator/RAM FIFO/Pilot Generator ==
  trigger : Inport
  Pilot Block Length Valid Generator : MATLAB Function  TreatAsAtomicUnit=on
  Pilot or Unmodulated Carrier : Constant  Value=fi(exp(1i*pi/4),1,18,16)  SampleTime=1/Rsym
  dataOut : Outport
  endOut : Outport  Port=2
  validOut : Outport  Port=3
  endOut1 : Outport  Port=4
  wires:
  Pilot Block Length Valid Generator/2(endOutm1) -> endOut1/1
  Pilot Block Length Valid Generator/3(validOut) -> validOut/1
  Pilot Block Length Valid Generator/1(endOut) -> endOut/1
  Pilot or Unmodulated Carrier/1 -> dataOut/1
  trigger/1 -> Pilot Block Length Valid Generator/1(trigger)

== system dvbs2hdlTransmitterCore/DVB-S2 Tx/BB Frame Generator/BB Header and Data CRC Generator/Data Field Generator/Continuous Streams ==
  dataIn : Inport
  validIn : Inport  Port=2
  frameEnd : Inport  Port=3
  frameStart : Inport  Port=4
  Delay{,1..3} (4 alike) : Delay  DelayLength=8+1+10
  dataOut : Outport
  validOut : Outport  Port=2
  frameEndOut : Outport  Port=3
  frameStartOut : Outport  Port=4
  wires:
  validIn/1 -> Delay1/1
  frameEnd/1 -> Delay2/1
  Delay2/1 -> frameEndOut/1
  Delay3/1 -> frameStartOut/1
  frameStart/1 -> Delay3/1
  Delay1/1 -> validOut/1
  dataIn/1 -> Delay/1
  Delay/1 -> dataOut/1

== system dvbs2hdlTransmitterCore/DVB-S2 Tx/BB Frame Generator/BB Header and Data CRC Generator/Data Field Generator/Packetized Streams ==
  dataIn : Inport
  startIn : Inport  Port=2
  endIn : Inport  Port=3
  validIn : Inport  Port=4
  frameEnd : Inport  Port=5
  frameStart : Inport  Port=6
  Delay : Delay  DelayLength=1
  Delay1 : Delay  DelayLength=1
  Delay2 : Delay  DelayLength=8
  Delay3 : Delay  DelayLength=10
  Delay4 : Delay  DelayLength=10
  Discard SYNC : MATLAB Function  TreatAsAtomicUnit=on
  MATLAB Function : MATLAB Function  TreatAsAtomicUnit=on
  Terminator : Terminator
  Terminator1 : Terminator
  User Packet CRC Generator : commhdlcrc/General CRC Generator HDL Optimized  Polynomial=[1 1 1 0 1 0 1 0 1]  InitialState=0  DirectMethod=off  ReflectInput=off  ReflectCRCChecksum=off  FinalXORValue=0  SimulateUsing=Code generation
  pktBits : Outport
  pktValid : Outport  Port=2
  frameEndOut : Outport  Port=3
  frameStartOut : Outport  Port=4
  wires:
  Delay4/1 -> MATLAB Function/2(frameEndIn)
  User Packet CRC Generator/4 -> pktValid/1
  Delay3/1 -> frameStartOut/1
  endIn/1 -> Discard SYNC/3(endIn)
  startIn/1 -> Discard SYNC/2(startIn)
  frameEnd/1 -> Delay/1
  frameStart/1 -> Delay2/1
  User Packet CRC Generator/1 -> pktBits/1
  Delay1/1 -> Delay3/1
  Discard SYNC/2(startOut) -> User Packet CRC Generator/2
  Discard SYNC/3(endOut) -> User Packet CRC Generator/3
  User Packet CRC Generator/2 -> Terminator/1
  User Packet CRC Generator/3 -> MATLAB Function/1(pktEndIn), Terminator1/1
  Discard SYNC/4(validOut) -> User Packet CRC Generator/4
  dataIn/1 -> Discard SYNC/1(dataIn)
  validIn/1 -> Discard SYNC/4(validIn)
  Delay/1 -> Delay4/1
  Delay2/1 -> Delay1/1
  MATLAB Function/1(frameEndOut) -> frameEndOut/1
  Discard SYNC/1(dataOut) -> User Packet CRC Generator/1

== system dvbs2hdlTransmitterCore/DVB-S2 Tx/BB Frame Generator/BB Header and Data CRC Generator/No HDL/No HDL ==
  rdy : Inport
  vld : Inport  Port=2
  Assertion : Assertion
  Logical Operator : Logic  AllPortsSameDT=off  OutDataTypeStr=boolean
  Logical Operator1 : Logic  Operator=NOT  AllPortsSameDT=off  OutDataTypeStr=boolean
  Logical Operator2 : Logic  Operator=NOT  AllPortsSameDT=off  OutDataTypeStr=boolean
  wires:
  Logical Operator2/1 -> Assertion/1
  rdy/1 -> Logical Operator1/1
  Logical Operator/1 -> Logical Operator2/1
  vld/1 -> Logical Operator/2
  Logical Operator1/1 -> Logical Operator/1

== system dvbs2hdlTransmitterCore/DVB-S2 Tx/BB Frame Generator/Data Store FIFO/No HDL/No HDL ==
  wr : Inport
  full : Inport  Port=2
  ncount : Inport  Port=3
  empty : Inport  Port=4
  rd : Inport  Port=5
  Assertion : Assertion  AssertionFailFcn=warning('push on to a full RAM');  StopWhenAssertionFail=off
  Assertion1 : Assertion  AssertionFailFcn=warning('pop from an empty RAM');  StopWhenAssertionFail=off
  Assertion2 : Assertion  AssertionFailFcn='count exceeded 80'
  Compare To Constant : simulink/Logic and Bit Operations/Compare To Constant  relop=<=  const=80  OutDataTypeStr=boolean
  Display : Display
  Logical Operator : Logic  Operator=NAND  AllPortsSameDT=off  OutDataTypeStr=boolean
  Logical Operator1 : Logic  Operator=NAND  AllPortsSameDT=off  OutDataTypeStr=boolean
  wires:
  Logical Operator1/1 -> Assertion1/1
  wr/1 -> Logical Operator/1
  full/1 -> Logical Operator/2
  ncount/1 -> Compare To Constant/1, Display/1
  empty/1 -> Logical Operator1/1
  Logical Operator/1 -> Assertion/1
  rd/1 -> Logical Operator1/2
  Compare To Constant/1 -> Assertion2/1

== system dvbs2hdlTransmitterCore/DVB-S2 Tx/FEC Encoder/DVB-S2 BCH Encoder/Parity Generation/Store and Retrieve Parity ==
  iwr_data : Inport  Partition=on  PartitionDimension=1  PartitionWidth=1  PartitionOffset=0
  iwr_addr : Inport  Port=2
  iwr_enb : Inport  Port=3  Partition=on  PartitionDimension=1  PartitionWidth=1  PartitionOffset=0
  ird_addr : Inport  Port=4
  For Each : ForEach  DisableCoverage=on
  parity RAM : hdlsllib/HDL RAMs/Simple Dual Port RAM  ram_size=3
  ird_data : Outport  ConcatenationDimension=1
  wires:
  ird_addr/1 -> parity RAM/4
  iwr_data/1 -> parity RAM/1
  iwr_addr/1 -> parity RAM/2
  iwr_enb/1 -> parity RAM/3
  parity RAM/1 -> ird_data/1

== system dvbs2hdlTransmitterCore/DVB-S2 Tx/Interleaver/DVB-S2 HDL Interleaver/RAM/Single RAM Using Two RAMs ==
  wr_din : Inport
  wr_addr : Inport  Port=2
  wr_en : Inport  Port=3
  rd_addr : Inport  Port=4
  Delay : Delay  DelayLength=1
  Extract Bits : simulink/Logic and Bit Operations/Extract Bits  bitsToExtract=Range of bits  numBits=8  bitIdxRange=[0 15]  outScalingMode=Treat bit field as an integer
  Extract Bits1 : simulink/Logic and Bit Operations/Extract Bits  bitsToExtract=Range of bits  numBits=8  bitIdxRange=16  outScalingMode=Treat bit field as an integer
  Extract Bits2 : simulink/Logic and Bit Operations/Extract Bits  bitsToExtract=Range of bits  numBits=8  bitIdxRange=[0 15]  outScalingMode=Treat bit field as an integer
  Extract Bits3 : simulink/Logic and Bit Operations/Extract Bits  bitsToExtract=Range of bits  numBits=8  bitIdxRange=16  outScalingMode=Treat bit field as an integer
  Logical Operator1 : Logic  Operator=NOT  AllPortsSameDT=off  OutDataTypeStr=boolean
  Logical Operator2 : Logic  AllPortsSameDT=off  OutDataTypeStr=boolean
  Logical Operator3 : Logic  AllPortsSameDT=off  OutDataTypeStr=boolean
  Multiport Switch : MultiPortSwitch  DataPortOrder=Zero-based contiguous  Inputs=2  zeroidx=on  SaturateOnIntegerOverflow=off  InputSameDT=off
  Simple Dual Port RAM : hdlsllib/HDL RAMs/Simple Dual Port RAM  ram_size=nextpow2(ConfigRx.RAMCapacity/2)
  Simple Dual Port RAM1 : hdlsllib/HDL RAMs/Simple Dual Port RAM  ram_size=nextpow2(ConfigRx.RAMCapacity/2)
  rd_dout : Outport
  wires:
  Delay/1 -> Multiport Switch/1
  Multiport Switch/1 -> rd_dout/1
  Simple Dual Port RAM1/1 -> Multiport Switch/3
  Extract Bits3/1 -> Delay/1
  Extract Bits2/1 -> Simple Dual Port RAM1/4, Simple Dual Port RAM/4
  Logical Operator2/1 -> Simple Dual Port RAM1/3
  Logical Operator3/1 -> Simple Dual Port RAM/3
  Logical Operator1/1 -> Logical Operator3/1
  Extract Bits1/1 -> Logical Operator2/1, Logical Operator1/1
  Extract Bits/1 -> Simple Dual Port RAM1/2, Simple Dual Port RAM/2
  Simple Dual Port RAM/1 -> Multiport Switch/2
  wr_din/1 -> Simple Dual Port RAM/1, Simple Dual Port RAM1/1
  rd_addr/1 -> Extract Bits3/1, Extract Bits2/1
  wr_en/1 -> Logical Operator2/2, Logical Operator3/2
  wr_addr/1 -> Extract Bits1/1, Extract Bits/1

== system dvbs2hdlTransmitterCore/DVB-S2 Tx/Interleaver/DVB-S2 HDL Interleaver/RAM/Wrap Address ==
  u : Inport
  Add : Sum  Inputs=+-  OutDataTypeStr=Inherit: Same as first input
  Compare To Constant : simulink/Logic and Bit Operations/Compare To Constant  relop=>=  const=ConfigRx.RAMCapacity  OutDataTypeStr=boolean
  Constant : Constant  Value=ConfigRx.RAMCapacity  OutDataTypeStr=Inherit: Inherit via back propagation  SampleTime=Tsamp
  Constant1 : Constant  Value=0  OutDataTypeStr=Inherit: Inherit via back propagation  SampleTime=Tsamp
  Data Type Duplicate : DataTypeDuplicate
  Data Type Duplicate1 : DataTypeDuplicate
  Data Type Conversion : DataTypeConversion  OutDataTypeStr=fixdt(0,nextpow2(ConfigRx.RAMCapacity),0)  SaturateOnIntegerOverflow=off  RndMeth=Floor
  Switch : Switch  Criteria=u2 ~= 0  SaturateOnIntegerOverflow=off  InputSameDT=off
  Switch1 : Switch  Criteria=u2 ~= 0  SaturateOnIntegerOverflow=off  InputSameDT=off
  y : Outport
  wires:
  u/1 -> Switch/3, Data Type Duplicate/1, Add/1, Compare To Constant/1
  Switch/1 -> Data Type Conversion/1
  Compare To Constant/1 -> Switch1/2, Switch/2
  Add/1 -> Switch/1
  Constant/1 -> Switch1/1, Data Type Duplicate1/1, Data Type Duplicate/2
  Data Type Conversion/1 -> y/1
  Switch1/1 -> Add/2
  Constant1/1 -> Data Type Duplicate1/2, Switch1/3

== system dvbs2hdlTransmitterCore/DVB-S2 Tx/Interleaver/DVB-S2 HDL Interleaver/RAM Address Generator/Generate and Add Read Base Address ==
  readAddrIn : Inport
  readValidIn : Inport  Port=2
  startIn : Inport  Port=3
  endIn : Inport  Port=4
  Add : Sum  Inputs=|++
  Delay{,1,3..4,18} (5 alike) : Delay  DelayLength=1
  Delay{5..9,11,13..16,19..20} (12 alike) : Delay
  Gain : Gain  Gain=ConfigRx.ShortFrameLen  ParamDataTypeStr=fixdt(0,nextpow2(16200),0)
  HDL Counter : hdlsllib/Sources/HDL Counter  CountType=Count limited  CountInit=0  CountStep=1  CountMax=(ConfigRx.RAMCapacity/ConfigRx.ShortFrameLen) - 1  CountFromType=Initial value  CountFrom=0  CountResetPort=off  CountLoadPort=off  CountEnbPort=on  CountDirPort=off  CountHitOutputPort=off  CountDataType=Unsigned  CountWordLen=nextpow2((ConfigRx.RAMCapacity/ConfigRx.ShortFrameLen) - 1)  CountFracLen=0  CountSampTime=1
  Indicate End of Every ShortFrame Length Samples : Subsystem
  Logical Operator : Logic  AllPortsSameDT=off  OutDataTypeStr=boolean
  No HDL Read Address Debug Scope : Subsystem
      settings: PortSchema="{\"entries\":[{\"content\":{\"sides\":[{\"content\":{\"connectorIds\":[]},\"type\":\"ConnectorPlacement.EquallySpacedRectSide\",\"uuid\":\"46203939-3922-41f1-8ac4-248045cc482a\"},{\"content\":{\"connectorIds\":[],\"side\":\"RIGHT\"},\"type\":\"ConnectorPlacement.EquallySpacedRectSide\",\"uuid\":\"e2b32fd8-ba43-4add-9433-a5e10ef1a6cd\"},{\"content\":{\"connectorIds\":[],\"side\":\"TOP\"},\"type\":\"ConnectorPlacement.EquallySpacedRectSide\",\"uuid\":\"bfa555b4-8f13-4832-b51a-da5c9f2f7d4d\"},{\"content\":{\"connectorIds\":[\"In1\",\"In2\",\"In3\",\"In4\"],\"side\":\"BOTTOM\"},\"type\":\"ConnectorPlacement.EquallySpacedRectSide\",\"uuid\":\"1df13975-2c0e-47d4-aefc-7a99adf3a0bb\"}]},\"type\":\"ConnectorPlacement.EquallySpacedConnector\",\"uuid\":\"18a89938-2c8d-49b5-957c-22a1a70f8f87\"}],\"packageUris\":[\"http://schema.mathworks.com/mf0/Connector/R2020b\"],\"version\":\"1.0\"}"
  Unit Delay Enabled Synchronous3 : hdlsllib/Discrete/Unit Delay Enabled Synchronous  InitialCondition=0.0  SampleTime=-1
  readAddrOut : Outport
  readValidOut : Outport  Port=2
  readStartOut : Outport  Port=3
  readEndOut : Outport  Port=4
  wires:
  Gain/1 -> Delay6/1
  Indicate End of Every ShortFrame Length Samples/1(endIndicate) -> Logical Operator/1
  readAddrIn/1 -> Indicate End of Every ShortFrame Length Samples/1(readAddr), Delay3/1
  HDL Counter/1 -> Delay5/1, No HDL Read Address Debug Scope/1(baseAddrIdx)
  Logical Operator/1 -> HDL Counter/1
  Unit Delay Enabled Synchronous3/1 -> Add/2
  Add/1 -> readAddrOut/1, No HDL Read Address Debug Scope/4(basePlusOffsetAddr)
  readValidIn/1 -> Logical Operator/2, Delay4/1
  endIn/1 -> Delay1/1, Delay/1
  Delay/1 -> Delay7/1
  Delay1/1 -> Delay9/1
  Delay3/1 -> Delay13/1
  Delay4/1 -> Delay14/1
  Delay5/1 -> Gain/1
  Delay6/1 -> Unit Delay Enabled Synchronous3/1
  Delay7/1 -> Delay8/1, No HDL Read Address Debug Scope/2(captureBaseAddrIdx)
  Delay8/1 -> Unit Delay Enabled Synchronous3/2
  Delay9/1 -> Delay11/1
  Delay11/1 -> readEndOut/1
  Delay13/1 -> Delay15/1
  Delay14/1 -> Delay16/1
  Delay15/1 -> Add/1, No HDL Read Address Debug Scope/3(offsetAddr)
  Delay16/1 -> readValidOut/1
  startIn/1 -> Delay18/1
  Delay18/1 -> Delay19/1
  Delay19/1 -> Delay20/1
  Delay20/1 -> readStartOut/1
